simulink model "Simulation_P1_r2023a"  (R2023a)
settings: Solver=FixedStepAuto  StartTime=0.0  StopTime=10  FixedStep=1e-3  RelTol=1e-3  EnableMultiTasking=on
undefined symbols (not defined in the file): D0, D1, D10, D11, D12, D13, D2, D3, D4, D5, D6, D7, D8, D9, PTA0, PTA1, PTA2, PTB23, PTB9, PTC16, PTC17, PTC2, PTC3, PTC4, PTD0, PTD1, PTD2, PTD3
libraries: frdmk64flib x15
settings Model: ExtModeTrigDuration=5  Creator=sherr  LastModifiedBy=mylyf
settings OptimizationCC: EnhancedBackFolding=on  PassReuseOutputArgsAs=Individual arguments  ZeroExternalMemoryAtStartup=off  ZeroInternalMemoryAtStartup=off  MaxStackSize=64  OptimizeBlockOrder=speed  DifferentSizesBufferReuse=on  OptimizationCustomize=off  EfficientTunableParamExpr=on
settings DebuggingCC: ParameterTunabilityLossMsg=error
settings HardwareCC: ProdBitPerPointer=32  ProdBitPerSizeT=32  ProdBitPerPtrDiffT=32  ProdLargestAtomicInteger=Long  ProdLargestAtomicFloat=Double  ProdWordSize=32  ProdHWDeviceType=ARM Compatible->ARM Cortex
settings SFSimCC: MATLABDynamicMemAlloc=off
settings RTWCC: Description=Embedded Coder  SystemTargetFile=ert.tlc  HardwareBoard=NXP FRDM-K64F  TLCOptions="-aInlineSetEventsForThisBaseRateFcn=TLC_FALSE -aSuppressMultiTaskScheduler=TLC_FALSE  -aRateBasedStepFcn=0"  TemplateMakefile=ert_default_tmf  Toolchain=GNU Tools for ARM Embedded Processors
settings CodeAppCC: ForceParamTrailComments=on  IgnoreCustomStorageClasses=off  OperatorAnnotations=on  SimulinkDataObjDesc=on  SFDataObjDesc=on  InsertBlockDesc=on
settings ERTTargetCC: ExtModeTransport=4  ExtModeMexFile=sendToCommService

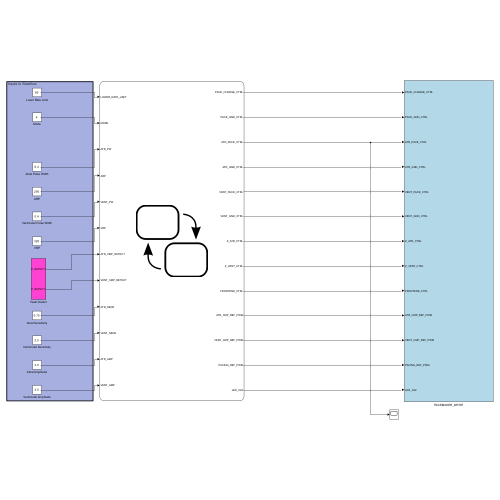
[thumbnail: Simulink's stored preview of the top-level diagram]
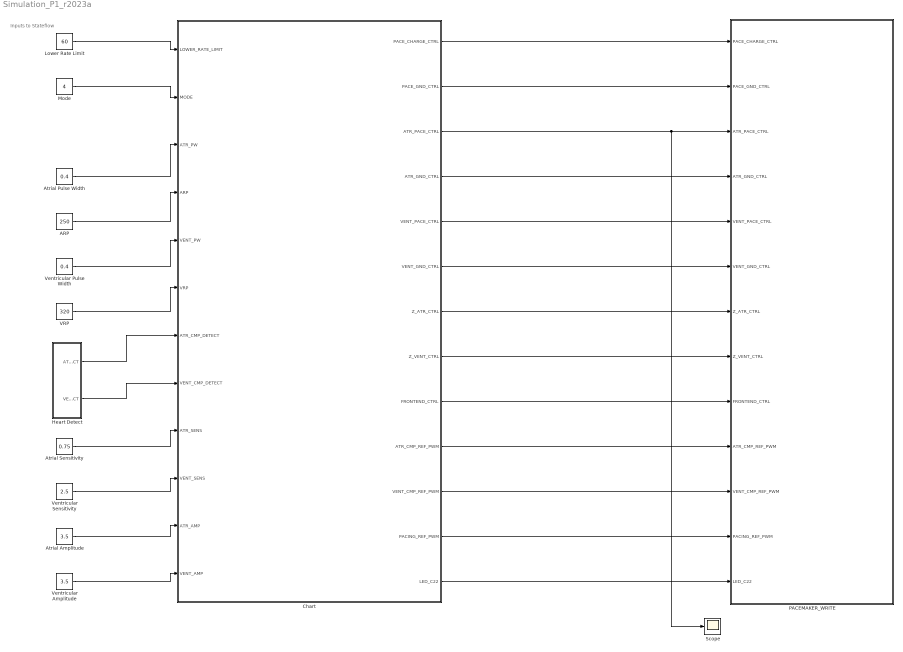
== system Simulation_P1_r2023a ==
  note: Inputs to Stateflow
  ARP : Constant  Value=250  OutDataTypeStr=uint16
  Atrial Amplitude : Constant  Value=3.5  OutDataTypeStr=double
  Atrial Pulse Width : Constant  Value=0.4  OutDataTypeStr=double
  Atrial Sensitivity : Constant  Value=0.75  OutDataTypeStr=double
  Chart : Stateflow chart  TreatAsAtomicUnit=on
  Heart Detect : Subsystem
  Lower Rate Limit : Constant  Value=60  OutDataTypeStr=uint16
  Mode : Constant  Value=4  OutDataTypeStr=uint16
  PACEMAKER_WRITE : Subsystem
  Scope : Scope
  VRP : Constant  Value=320  OutDataTypeStr=uint16
  Ventricular Amplitude : Constant  Value=3.5  OutDataTypeStr=double
  Ventricular Pulse Width : Constant  Value=0.4  OutDataTypeStr=double
  Ventricular Sensitivity : Constant  Value=2.5  OutDataTypeStr=double
  wires:
  Chart/10(ATR_CMP_REF_PWM) -> PACEMAKER_WRITE/10(ATR_CMP_REF_PWM)
  ARP/1 -> Chart/4(ARP)
  Chart/8(Z_VENT_CTRL) -> PACEMAKER_WRITE/8(Z_VENT_CTRL)
  Chart/1(PACE_CHARGE_CTRL) -> PACEMAKER_WRITE/1(PACE_CHARGE_CTRL)
  Chart/7(Z_ATR_CTRL) -> PACEMAKER_WRITE/7(Z_ATR_CTRL)
  Heart Detect/2(VENT_CMP_DETECT) -> Chart/8(VENT_CMP_DETECT)
  Chart/5(VENT_PACE_CTRL) -> PACEMAKER_WRITE/5(VENT_PACE_CTRL)
  Chart/11(VENT_CMP_REF_PWM) -> PACEMAKER_WRITE/11(VENT_CMP_REF_PWM)
  Chart/9(FRONTEND_CTRL) -> PACEMAKER_WRITE/9(FRONTEND_CTRL)
  Chart/6(VENT_GND_CTRL) -> PACEMAKER_WRITE/6(VENT_GND_CTRL)
  Chart/4(ATR_GND_CTRL) -> PACEMAKER_WRITE/4(ATR_GND_CTRL)
  Chart/12(PACING_REF_PWM) -> PACEMAKER_WRITE/12(PACING_REF_PWM)
  Ventricular Amplitude/1 -> Chart/12(VENT_AMP)
  Ventricular Pulse Width/1 -> Chart/5(VENT_PW)
  VRP/1 -> Chart/6(VRP)
  Atrial Pulse Width/1 -> Chart/3(ATR_PW)
  Atrial Sensitivity/1 -> Chart/9(ATR_SENS)
  Mode/1 -> Chart/2(MODE)
  Ventricular Sensitivity/1 -> Chart/10(VENT_SENS)
  Chart/3(ATR_PACE_CTRL) -> Scope/1, PACEMAKER_WRITE/3(ATR_PACE_CTRL)
  Heart Detect/1(ATR_CMP_DETECT) -> Chart/7(ATR_CMP_DETECT)
  Lower Rate Limit/1 -> Chart/1(LOWER_RATE_LIMIT)
  Atrial Amplitude/1 -> Chart/11(ATR_AMP)
  Chart/2(PACE_GND_CTRL) -> PACEMAKER_WRITE/2(PACE_GND_CTRL)
  Chart/13(LED_C22) -> PACEMAKER_WRITE/13(LED_C22)

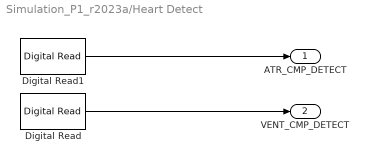
== system Simulation_P1_r2023a/Heart Detect ==
  Digital Read : frdmk64flib/Digital Read  Whichpin=PTC17 (D1)  SampleTime=-1
  Digital Read1 : frdmk64flib/Digital Read  Whichpin=PTC16 (D0)  SampleTime=-1
  ATR_CMP_DETECT : Outport
  VENT_CMP_DETECT : Outport  Port=2
  wires:
  Digital Read/1 -> VENT_CMP_DETECT/1
  Digital Read1/1 -> ATR_CMP_DETECT/1

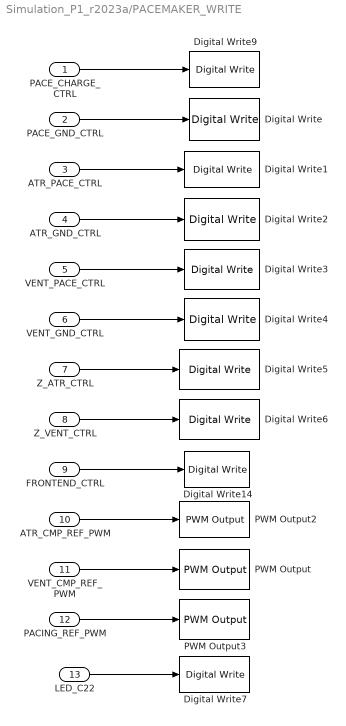
== system Simulation_P1_r2023a/PACEMAKER_WRITE ==
  PACE_CHARGE_CTRL : Inport
  PACE_GND_CTRL : Inport  Port=2
  ATR_PACE_CTRL : Inport  Port=3
  ATR_GND_CTRL : Inport  Port=4
  VENT_PACE_CTRL : Inport  Port=5
  VENT_GND_CTRL : Inport  Port=6
  Z_ATR_CTRL : Inport  Port=7
  Z_VENT_CTRL : Inport  Port=8
  FRONTEND_CTRL : Inport  Port=9
  ATR_CMP_REF_PWM : Inport  Port=10
  VENT_CMP_REF_PWM : Inport  Port=11
  PACING_REF_PWM : Inport  Port=12
  LED_C22 : Inport  Port=13
  Digital Write : frdmk64flib/Digital Write  Whichpin=PTD0 (D10)
  Digital Write1 : frdmk64flib/Digital Write  Whichpin=PTA0 (D8)
  Digital Write14 : frdmk64flib/Digital Write  Whichpin=PTD1 (D13)
  Digital Write2 : frdmk64flib/Digital Write  Whichpin=PTD2 (D11)
  Digital Write3 : frdmk64flib/Digital Write  Whichpin=PTC4 (D9)
  Digital Write4 : frdmk64flib/Digital Write  Whichpin=PTD3 (D12)
  Digital Write5 : frdmk64flib/Digital Write  Whichpin=PTB23 (D4)
  Digital Write6 : frdmk64flib/Digital Write  Whichpin=PTC3 (D7)
  Digital Write7 : frdmk64flib/Digital Write  Whichpin=BLUE_LED
  Digital Write9 : frdmk64flib/Digital Write  Whichpin=PTB9 (D2)
  PWM Output : frdmk64flib/PWM Output  Whichpin=PTA1 (D3)  InitialFrequency=2000  InitialDutyCycle=100
  PWM Output2 : frdmk64flib/PWM Output  Whichpin=PTC2 (D6)  InitialFrequency=2000  InitialDutyCycle=100
  PWM Output3 : frdmk64flib/PWM Output  Whichpin=PTA2 (D5)  InitialFrequency=2000  InitialDutyCycle=100
  wires:
  PACE_GND_CTRL/1 -> Digital Write/1
  ATR_CMP_REF_PWM/1 -> PWM Output2/1
  Z_ATR_CTRL/1 -> Digital Write5/1
  ATR_GND_CTRL/1 -> Digital Write2/1
  Z_VENT_CTRL/1 -> Digital Write6/1
  FRONTEND_CTRL/1 -> Digital Write14/1
  PACE_CHARGE_CTRL/1 -> Digital Write9/1
  VENT_GND_CTRL/1 -> Digital Write4/1
  PACING_REF_PWM/1 -> PWM Output3/1
  ATR_PACE_CTRL/1 -> Digital Write1/1
  VENT_CMP_REF_PWM/1 -> PWM Output/1
  VENT_PACE_CTRL/1 -> Digital Write3/1
  LED_C22/1 -> Digital Write7/1

== stateflow chart Simulation_P1_r2023a/Chart ==
  state AOO [group]
    state CHARGING
      entry:
      %Begin Charging C22 Capacitor
      ATR_PACE_CTRL = 0
      VENT_PACE_CTRL = 0
      PACING_REF_PWM = 100*ATR_AMP/5
      PACE_CHARGE_CTRL = 1
      %Begin Discharging C21 Blocking Capacitor
      PACE_GND_CTRL = 1
      VENT_PACE_CTRL = 0
      Z_ATR_CTRL = 0
      Z_VENT_CTRL = 0
      ATR_PACE_CTRL = 0
      ATR_GND_CTRL = 1
      VENT_GND_CTRL = 0
      %Test
      LED_C22 = 1
    state DISCHARGING
      entry:
      %Discharge C22 into Atrium (AtrialPacing)
      %Begin Charging C21 Blocking Capacitor
      PACE_CHARGE_CTRL = 0
      PACE_GND_CTRL = 1
      ATR_PACE_CTRL = 1
      ATR_GND_CTRL = 0
      Z_ATR_CTRL = 0
      Z_VENT_CTRL = 0
      VENT_GND_CTRL = 0
      VENT_PACE_CTRL  = 0
    AOO.CHARGING -> AOO.DISCHARGING [order 1] : [after(((60000/LOWER_RATE_LIMIT)-ATR_PW), msec)]
    AOO.DISCHARGING -> AOO.CHARGING : [after(ATR_PW, msec)]
  state AAI [group]
    state PROXY
      entry:
      %Discharge C21 Blocking Capacitor
      PACE_GND_CTRL = true;
      VENT_PACE_CTRL = false;
      Z_ATR_CTRL = false;
      Z_VENT_CTRL = false;
      ATR_PACE_CTRL = false;
      ATR_GND_CTRL = true;
      VENT_GND_CTRL = false;
      %Charge C22
      ATR_PACE_CTRL = false;
      VENT_PACE_CTRL = false;
      PACING_REF_PWM = 100*ATR_AMP/5;
      PACE_CHARGE_CTRL = true;
    state CHARGING
      entry:
      %Sensing Circuitry
      FRONTEND_CTRL = HIGH
      %Assume appropriate PWM threshold
      ATR_CMP_REF_PWM = 100*ATR_AMP/5;
      VENT_CMP_REF_PWM = 0
      %Begin Charging C22 Capacitor
      ATR_PACE_CTRL = false;
      VENT_PACE_CTRL = false;
      PACING_REF_PWM = 100*ATR_AMP/5;
      PACE_CHARGE_CTRL = true;
      %Begin Discharging C21 Blocking Capacitor
      PACE_GND_CTRL = true;
      VENT_PACE_CTRL = false;
      Z_ATR_CTRL = false;
      Z_VENT_CTRL = false;
      ATR_PACE_CTRL = false;
      ATR_GND_CTRL = true;
      VENT_GND_CTRL = false;
    state DISCHARGING
      entry:
      %Discharge C22 into Atrium (Atrial Pacing)
      %Begin Charging Blocking Capacitor
      PACE_CHARGE_CTRL = LOW
      PACE_GND_CTRL = HIGH
      ATR_PACE_CTRL = HIGH
      ATR_GND_CTRL = LOW
      Z_ATR_CTRL = LOW
      Z_VENT_CTRL = LOW
      VENT_GND_CTRL = LOW
      VENT_PACE_CTRL  = LOW
    AAI.DISCHARGING -> AAI.PROXY : [after(ATR_PW, msec)]
    AAI.PROXY -> AAI.CHARGING : [after(ARP, msec)]
    (junction 116) -> AAI.PROXY : [after(LOWER_RATE_LIMIT, msec)]
    AAI.CHARGING -> (junction 116) [order 1] : [ATR_CMP_DETECT == HIGH]
    AAI.CHARGING -> AAI.DISCHARGING [order 2] : after(((60000/LOWER_RATE_LIMIT)-ATR_PW), msec)[ATR_CMP_DETECT == LOW]
  state INITIAL
    %Initial State
  state VOO [group]
    state CHARGING
      entry:
      %Begin Charging C22 Capacitor
      ATR_PACE_CTRL = false;
      VENT_PACE_CTRL = false;
      PACING_REF_PWM = 100*VENT_AMP/5
      PACE_CHARGE_CTRL = true;
      %Begin Discharging C21 Blocking Capacitor
      PACE_GND_CTRL = true;
      VENT_PACE_CTRL = false;
      Z_ATR_CTRL = false;
      Z_VENT_CTRL = false;
      ATR_PACE_CTRL = false;
      ATR_GND_CTRL = false;
      VENT_GND_CTRL = true;
    state DISCHARGING
      entry:
      %Discharge C22 into Ventricle (Vent Pacing)
      %Begin Charging Blocking Capacitor
      PACE_CHARGE_CTRL = false;
      PACE_GND_CTRL = true;
      ATR_PACE_CTRL = false;
      ATR_GND_CTRL = false;
      Z_ATR_CTRL = false;
      Z_VENT_CTRL = false;
      VENT_GND_CTRL = false;
      VENT_PACE_CTRL  = true;
    VOO.CHARGING -> VOO.DISCHARGING [order 1] : [after(((60000/LOWER_RATE_LIMIT)-VENT_PW), msec)]
    VOO.DISCHARGING -> VOO.CHARGING : [after(VENT_PW, msec)]
  state VVI [group]
    state PROXY
      entry:
      %Step 1
      %Discharge C21 Blocking Capacitor
      PACE_GND_CTRL = HIGH
      VENT_PACE_CTRL = LOW
      Z_ATR_CTRL = LOW
      Z_VENT_CTRL = LOW
      ATR_PACE_CTRL = LOW
      ATR_GND_CTRL = LOW
      VENT_GND_CTRL = HIGH
      %Step 2
      %Charge C22
      ATR_PACE_CTRL = LOW
      VENT_PACE_CTRL = LOW
      PACING_REF_PWM = 100*VENT_AMP/5;
      PACE_CHARGE_CTRL = HIGH
    state CHARGING
      entry:
      %Sense Circuit
      FRONTEND_CTRL = true
      VENT_CMP_REF_PWM = (100*VENT_AMP)/5;
      ATR_CMP_REF_PWM = 0;
      %Begin Charging C22 Capacitor
      ATR_PACE_CTRL = LOW
      VENT_PACE_CTRL = LOW
      PACING_REF_PWM = 100*VENT_AMP/5;
      PACE_CHARGE_CTRL = HIGH
      %Begin Discharging Blocking Capacitor
      PACE_GND_CTRL = HIGH
      VENT_PACE_CTRL = LOW
      Z_ATR_CTRL = LOW
      Z_VENT_CTRL = LOW
      ATR_PACE_CTRL = LOW
      ATR_GND_CTRL = LOW
      VENT_GND_CTRL = HIGH
    state DISCHARGING
      entry:
      %Step 1:
      %Discharge C22 into Ventricle (Vent Pacing)
      %Begin Charging Blocking Capacitor
      PACE_CHARGE_CTRL = LOW
      PACE_GND_CTRL = HIGH
      ATR_PACE_CTRL = LOW
      ATR_GND_CTRL = LOW
      Z_ATR_CTRL = LOW
      Z_VENT_CTRL = LOW
      VENT_GND_CTRL = LOW
      VENT_PACE_CTRL  = HIGH
    VVI.DISCHARGING -> VVI.PROXY : [after(VENT_PW, msec)]
    VVI.PROXY -> VVI.CHARGING : [after(VRP, msec)]
    (junction 657) -> VVI.PROXY : [after(LOWER_RATE_LIMIT, msec)]
    VVI.CHARGING -> (junction 657) [order 1] : [VENT_CMP_DETECT ==  HIGH]
    VVI.CHARGING -> VVI.DISCHARGING [order 2] : after(((60000/LOWER_RATE_LIMIT)-VENT_PW), msec)[VENT_CMP_DETECT ==  LOW]
  INITIAL -> VVI.CHARGING [order 4] : [MODE == 4]
  AOO.CHARGING -> INITIAL [order 2] : [MODE ~= 1]
  AAI.CHARGING -> INITIAL [order 3] : [MODE ~= 2]
  VVI.CHARGING -> INITIAL [order 3] : [MODE ~= 4]
  INITIAL -> AOO.CHARGING [order 1] : [MODE == 1]
  INITIAL -> VOO.CHARGING [order 3] : [MODE == 3]
  INITIAL -> AAI.CHARGING [order 2] : [MODE == 2]
  VOO.CHARGING -> INITIAL [order 2] : [MODE ~= 3]
  (default) -> INITIAL
  data: PACE_CHARGE_CTRL output uint16; PACE_GND_CTRL output uint16; ATR_PACE_CTRL output uint16; ATR_GND_CTRL output uint16; VENT_PACE_CTRL output uint16; VENT_GND_CTRL output uint16; Z_ATR_CTRL output uint16; Z_VENT_CTRL output uint16; LOWER_RATE_LIMIT input uint16; MODE input uint16; ATR_PW input double; ARP input uint16; VENT_PW input double; VRP input uint16; HIGH local uint16 =1; LOW local uint16 =0; ATR_CMP_DETECT input boolean; VENT_CMP_DETECT input boolean; ATR_SENS input; VENT_SENS input; ATR_AMP input; VENT_AMP input; FRONTEND_CTRL output; ATR_CMP_REF_PWM output; VENT_CMP_REF_PWM output; PACING_REF_PWM output; LED_C22 output; true local uint16 =1; false local uint16 =0
